simulink model "LD_V1"  (R2019a)
settings: Solver=VariableStepAuto  StartTime=0.0  StopTime=10.0  RelTol=1e-3
model workspace (MAT data in the model file):
  FBv = [-0.360628002737 -0.359628002737 -0.358628002737 -0.357628002737 -0.356628002737 -0.355628002737 -0.354628002737 -0.353628002737 -0.352628002737 -0.351628002737 -0.350628002737 -0.349628002737 ... (3119 elements, 1x3119)]
  G_g = 16.59
  G_h = 8.17
  g = 9.81
  h_s = 0.5
  l = 2.8
  l_v = 1.344
  reifenX = [0 0.25 1]
  reifenY = [0 1 1]
  useController = 1
  v0 = 22.2222222222
  z_time = [0 1.5 1.95 2.15 10]
  z_vals = [0 0 0.1 1 1]
  zh_z = 1
  zv_z = 1
libraries: simulink x3
(part 1 of 2)
settings Model: Creator=Mel  LastModifiedBy=Mel
settings DataIOCC: ReturnWorkspaceOutputs=off
settings DebuggingCC: ArithmeticOperatorsInVariantConditions=warning

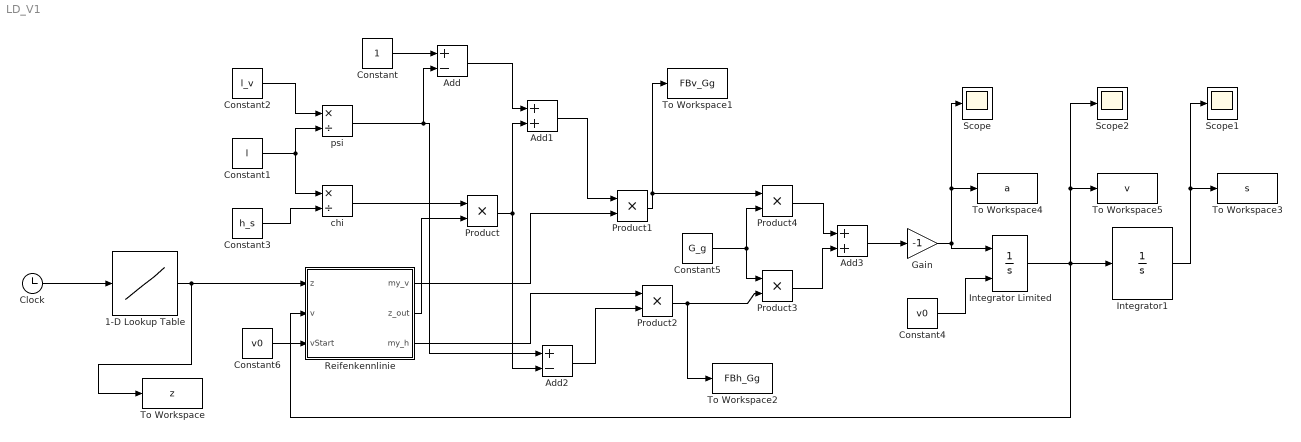
== system LD_V1 ==
  1-D Lookup Table : Lookup_n-D  NumberOfTableDimensions=1  BreakpointsForDimension1=z_time  Table=z_vals  InternalRulePriority=Speed  RndMeth=Simplest  InputSameDT=on
  Add : Sum  Inputs=+-
  Add1 : Sum
  Add2 : Sum  Inputs=+-
  Add3 : Sum
  Clock : Clock
  Constant : Constant
  Constant1 : Constant  Value=l
  Constant2 : Constant  Value=l_v
  Constant3 : Constant  Value=h_s
  Constant4 : Constant  Value=v0
  Constant5 : Constant  Value=G_g
  Constant6 : Constant  Value=v0
  Gain : Gain  Gain=-1
  Integrator Limited : Integrator  InitialConditionSource=external  LimitOutput=on  UpperSaturationLimit=100  LowerSaturationLimit=0
  Integrator1 : Integrator
  Product{,1..4} (5 alike) : Product
  Reifenkennlinie : Subsystem
  Scope : Scope
  Scope1 : Scope
  Scope2 : Scope
  To Workspace : ToWorkspace  VariableName=z  SaveFormat=Timeseries  SampleTime=-1
  To Workspace1 : ToWorkspace  VariableName=FBv_Gg  SaveFormat=Timeseries  SampleTime=-1
  To Workspace2 : ToWorkspace  VariableName=FBh_Gg  SaveFormat=Timeseries  SampleTime=-1
  To Workspace3 : ToWorkspace  VariableName=s  SaveFormat=Timeseries  SampleTime=-1
  To Workspace4 : ToWorkspace  VariableName=a  SaveFormat=Timeseries  SampleTime=-1
  To Workspace5 : ToWorkspace  VariableName=v  SaveFormat=Timeseries  SampleTime=-1
  chi : Product  Inputs=*/
  psi : Product  Inputs=*/
  wires:
  Clock/1 -> 1-D Lookup Table/1
  Constant3/1 -> chi/2
  Constant1/1 -> chi/1, psi/2
  Constant2/1 -> psi/1
  Constant/1 -> Add/1
  chi/1 -> Product/1
  Add/1 -> Add1/1
  Product/1 -> Add2/2, Add1/2
  Add1/1 -> Product1/1
  psi/1 -> Add2/1, Add/2
  Add2/1 -> Product2/2
  1-D Lookup Table/1 -> Reifenkennlinie/1(z), To Workspace/1
  Product2/1 -> To Workspace2/1, Product3/2
  Constant5/1 -> Product3/1, Product4/2
  Product1/1 -> To Workspace1/1, Product4/1
  Product4/1 -> Add3/1
  Product3/1 -> Add3/2
  Add3/1 -> Gain/1
  Gain/1 -> Integrator Limited/1, To Workspace4/1, Scope/1
  Constant4/1 -> Integrator Limited/2
  Integrator1/1 -> To Workspace3/1, Scope1/1
  Constant6/1 -> Reifenkennlinie/3(vStart)
  Integrator Limited/1 -> Reifenkennlinie/2(v), To Workspace5/1, Scope2/1, Integrator1/1
  Reifenkennlinie/1(my_v) -> Product1/2
  Reifenkennlinie/2(z_out) -> Product/2
  Reifenkennlinie/3(my_h) -> Product2/1

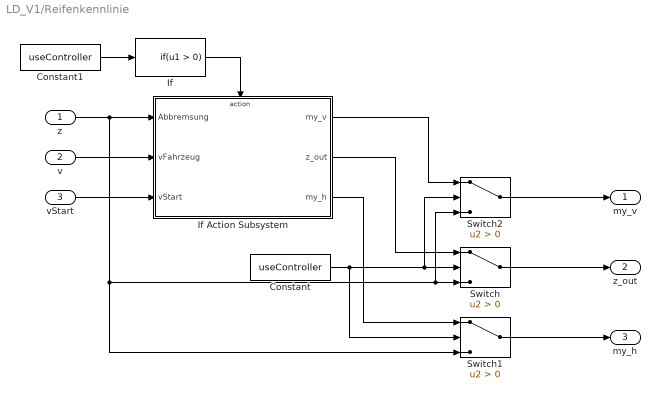
== system LD_V1/Reifenkennlinie ==
  z : Inport
  v : Inport  Port=2
  vStart : Inport  Port=3
  Constant : Constant  Value=useController
  Constant1 : Constant  Value=useController
  If : If  ShowElse=off
  If Action Subsystem : Subsystem  TreatAsAtomicUnit=on
  Switch : Switch  Criteria=u2 > Threshold
  Switch1 : Switch  Criteria=u2 > Threshold
  Switch2 : Switch  Criteria=u2 > Threshold
  my_v : Outport
  z_out : Outport  Port=2
  my_h : Outport  Port=3
  wires:
  z/1 -> Switch1/3, Switch2/3, Switch/3, If Action Subsystem/1(Abbremsung)
  v/1 -> If Action Subsystem/2(vFahrzeug)
  vStart/1 -> If Action Subsystem/3(vStart)
  Constant/1 -> Switch1/2, Switch2/2, Switch/2
  If Action Subsystem/2(z_out) -> Switch/1
  Switch/1 -> z_out/1
  Switch1/1 -> my_h/1
  If Action Subsystem/3(my_h) -> Switch1/1
  Switch2/1 -> my_v/1
  If Action Subsystem/1(my_v) -> Switch2/1
  Constant1/1 -> If/1
  If/1 -> If Action Subsystem/Action
